simulink model "Lab1_Challenge"  (R2020b)
settings: Solver=VariableStepAuto  StartTime=0.0  StopTime=0.25  RelTol=1e-3
undefined symbols (not defined in the file): C, D_w, degs2rpm, K, K_I, Kw, N_w, Nu, Nx, rpm2rads, sens, step_amplitude
settings Model: Creator=Musta  LastModifiedBy=Musta

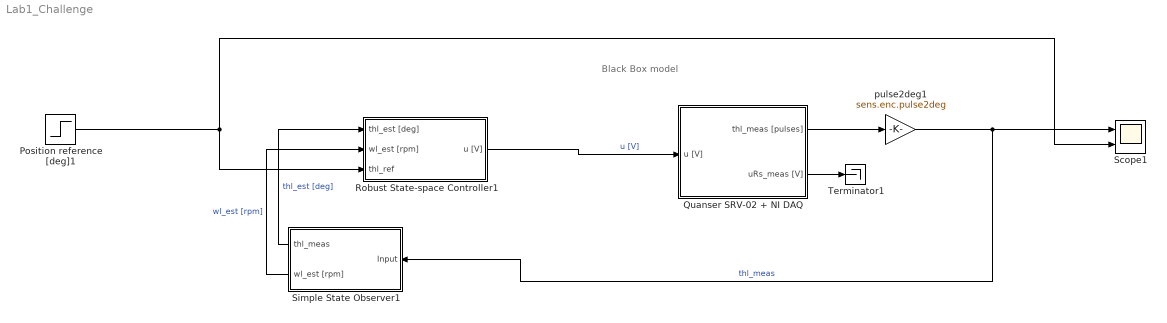
== system Lab1_Challenge ==
  note: Black Box model
  Position reference [deg]1 : Step  Time=0  After=step_amplitude  SampleTime=0
  Quanser SRV-02 + NI DAQ : Subsystem  mask(Quanser SRV-02 (with inertial load) + NI DAQ){Ts=0.001, fricType=Karnopp}
      mask prompts: Ts "NI DAQ Sample Time:"; fricType "Friction model"
      mask help: Quanser SRV-02 (with inertial load) + NI DAQ model.
      mask init:
      | %%  Sensors data
      | 
      | %   shunt resistor
      | sens.curr.Rs = 0.5;                         %   resistance [Ohm]   
      | sens.curr.uRs_std = 0.01;                   %   voltage noise standard dev [V]                           
      | sens.curr.uRs_var = sens.curr.uRs_std^2;	%   voltage noise variance [V^2]
      | 
      | %   Hewlett-Packard HEDS-5540#A06 optical encoder
      | sens.enc.ppr = 500*4;                       %   pulses per rotation
      | sens.enc.pulse2deg = 360/sens.enc.ppr;      %   [pulses] -> [deg]
      | sens.enc.pulse2rad = 2*pi/sens.enc.ppr;     %   [pulses] -> [rad]
      | sens.enc.deg2pulse = sens.enc.ppr/360;      %   [deg] -> [pulses]
      | sens.enc.rad2pulse = sens.enc.ppr/2/pi;     %   [rad] -> [pulses]
      | 
      | 
      | %%  Data acquisition board (daq) data
      | 
      | %   NI PCI-6221 DAC data
      | daq.dac.bits = 16;                                  %   resolution (bits)
      | daq.dac.fs   = 10;                                  %   full scale 
      | daq.dac.q    = 2*daq.dac.fs/(2^daq.dac.bits-1);     %	quantization
      | 
      | %   NI PCI-6221 ADC data
      | daq.adc.bits = 16;                                  %   resolution (bits)
      | daq.adc.fs   = 10;                                  %   full scale (as set in SLDRT Analog Input block)
      | daq.adc.q    = 2*daq.adc.fs/(2^daq.adc.bits-1);     %   quantization
      mask Help:
      | Riccardo Antonello (antonello@dei.unipd.it)
      | 
      | April 24, 2020
      | 
      | Dept. of Information Engineering, University of Padova
      mask TypeOptions fricType: Coulomb + viscous | Karnopp
  Robust State-space Controller1 : Subsystem
  Scope1 : Scope  NumInputPorts=2
  Simple State Observer1 : Subsystem
  Terminator1 : Terminator
  pulse2deg1 : Gain  Gain=sens.enc.pulse2deg
  wires:
  Simple State Observer1/1(thl_meas) -> Robust State-space Controller1/1(thl_est [deg])  "thl_est [deg]"
  Robust State-space Controller1/1(u [V]) -> Quanser SRV-02 + NI DAQ/1(u [V])  "u [V]"
  Quanser SRV-02 + NI DAQ/2(uRs_meas [V]) -> Terminator1/1
  Position reference [deg]1/1 -> Robust State-space Controller1/3(thl_ref), Scope1/2
  Simple State Observer1/2(wl_est [rpm]) -> Robust State-space Controller1/2(wl_est [rpm])  "wl_est [rpm]"
  pulse2deg1/1 -> Scope1/1, Simple State Observer1/1(Input)  "thl_meas"
  Quanser SRV-02 + NI DAQ/1(thl_meas [pulses]) -> pulse2deg1/1

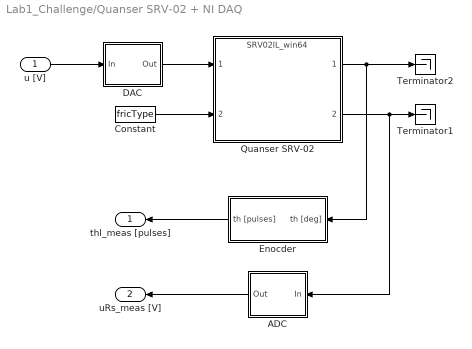
== system Lab1_Challenge/Quanser SRV-02 + NI DAQ ==
  u [V] : Inport
  ADC : Subsystem
  Constant : Constant  Value=fricType
  DAC : Subsystem
  Enocder : Subsystem
  Quanser SRV-02 : ModelReference  ModelNameDialog=SRV02IL_win64.slxp  ModelReferenceVersion=1.44  CopyOfModelProtected=on
  Terminator1 : Terminator
  Terminator2 : Terminator
  thl_meas [pulses] : Outport
  uRs_meas [V] : Outport  Port=2
  wires:
  Enocder/1(th [pulses]) -> thl_meas [pulses]/1
  ADC/1(Out) -> uRs_meas [V]/1
  DAC/1(Out) -> Quanser SRV-02/1
  Quanser SRV-02/2 -> ADC/1(In), Terminator1/1
  u [V]/1 -> DAC/1(In)
  Quanser SRV-02/1 -> Enocder/1(th [deg]), Terminator2/1
  Constant/1 -> Quanser SRV-02/2

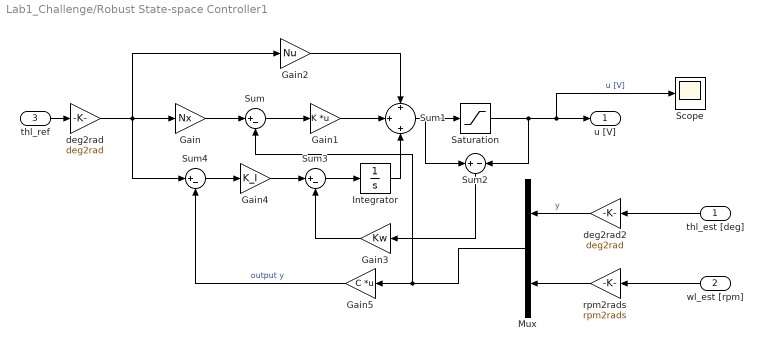
== system Lab1_Challenge/Robust State-space Controller1 ==
  thl_est [deg] : Inport
  wl_est [rpm] : Inport  Port=2
  thl_ref : Inport  Port=3
  Gain : Gain  Gain=Nx
  Gain1 : Gain  Gain=K  Multiplication=Matrix(K*u)
  Gain2 : Gain  Gain=Nu
  Gain3 : Gain  Gain=Kw
  Gain4 : Gain  Gain=K_I
  Gain5 : Gain  Gain=C  Multiplication=Matrix(K*u)
  Integrator : Integrator
  Mux : Mux  Inputs=2
  Saturation : Saturate  UpperLimit=10  LowerLimit=-10
  Scope : Scope
  Sum : Sum  Inputs=|+-
  Sum1 : Sum  Inputs=+|+|+
  Sum2 : Sum  Inputs=+|-
  Sum3 : Sum  Inputs=|+-
  Sum4 : Sum  Inputs=|+-
  deg2rad : Gain  Gain=deg2rad
  deg2rad2 : Gain  Gain=deg2rad
  rpm2rads : Gain  Gain=rpm2rads
  u [V] : Outport
  wires:
  Saturation/1 -> Sum2/2, u [V]/1, Scope/1  "u [V]"
  rpm2rads/1 -> Mux/2
  deg2rad2/1 -> Mux/1  "y"
  thl_est [deg]/1 -> deg2rad2/1
  wl_est [rpm]/1 -> rpm2rads/1
  thl_ref/1 -> deg2rad/1
  Gain/1 -> Sum/1
  Sum/1 -> Gain1/1
  Gain1/1 -> Sum1/2
  Gain2/1 -> Sum1/1
  Sum1/1 -> Saturation/1, Sum2/1
  Gain4/1 -> Sum3/1
  Sum4/1 -> Gain4/1
  deg2rad/1 -> Gain2/1, Sum4/1, Gain/1
  Integrator/1 -> Sum1/3
  Sum3/1 -> Integrator/1
  Gain3/1 -> Sum3/2
  Sum2/1 -> Gain3/1
  Mux/1 -> Sum/2, Gain5/1
  Gain5/1 -> Sum4/2  "output y"

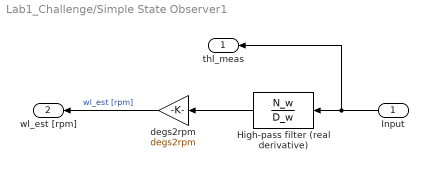
== system Lab1_Challenge/Simple State Observer1 ==
  Input : Inport
  High-pass filter (real derivative) : TransferFcn  Numerator=N_w  Denominator=D_w
  degs2rpm : Gain  Gain=degs2rpm
  thl_meas : Outport
  wl_est [rpm] : Outport  Port=2
  wires:
  Input/1 -> thl_meas/1, High-pass filter (real derivative)/1
  High-pass filter (real derivative)/1 -> degs2rpm/1
  degs2rpm/1 -> wl_est [rpm]/1  "wl_est [rpm]"

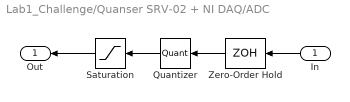
== system Lab1_Challenge/Quanser SRV-02 + NI DAQ/ADC ==
  In : Inport
  Quantizer : Quantizer  QuantizationInterval=daq.adc.q
  Saturation : Saturate  UpperLimit=daq.adc.fs  LowerLimit=-daq.adc.fs
  Zero-Order Hold : ZeroOrderHold  SampleTime=Ts
  Out : Outport
  wires:
  Saturation/1 -> Out/1
  In/1 -> Zero-Order Hold/1
  Quantizer/1 -> Saturation/1
  Zero-Order Hold/1 -> Quantizer/1

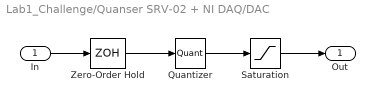
== system Lab1_Challenge/Quanser SRV-02 + NI DAQ/DAC ==
  In : Inport
  Quantizer : Quantizer  QuantizationInterval=daq.dac.q
  Saturation : Saturate  UpperLimit=daq.dac.fs  LowerLimit=-daq.dac.fs
  Zero-Order Hold : ZeroOrderHold  SampleTime=Ts
  Out : Outport
  wires:
  Quantizer/1 -> Saturation/1
  In/1 -> Zero-Order Hold/1
  Zero-Order Hold/1 -> Quantizer/1
  Saturation/1 -> Out/1

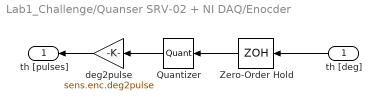
== system Lab1_Challenge/Quanser SRV-02 + NI DAQ/Enocder ==
  th [deg] : Inport
  Quantizer : Quantizer  QuantizationInterval=sens.enc.pulse2deg
  Zero-Order Hold : ZeroOrderHold  SampleTime=Ts
  deg2pulse : Gain  Gain=sens.enc.deg2pulse
  th [pulses] : Outport
  wires:
  Quantizer/1 -> deg2pulse/1
  th [deg]/1 -> Zero-Order Hold/1
  Zero-Order Hold/1 -> Quantizer/1
  deg2pulse/1 -> th [pulses]/1
